simulink model "KinovaBlockdiagram"  (R2022b)
settings: Solver=VariableStepAuto  StartTime=0.0  StopTime=10.0  RelTol=1e-3
undefined symbols (not defined in the file or in its folder): Admittance, forwardKinematics, K, M
settings Model: Creator=KCY  LastModifiedBy=KCY

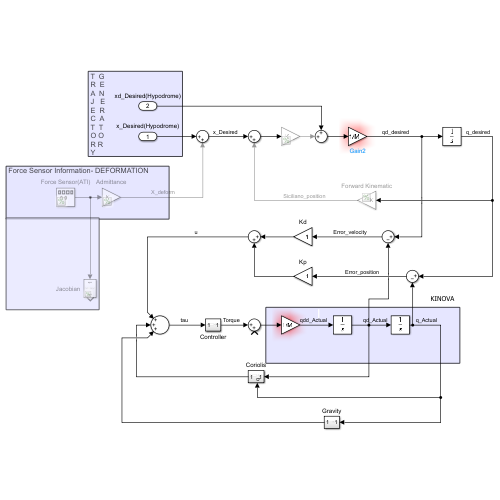
[thumbnail: Simulink's stored preview of the top-level diagram]
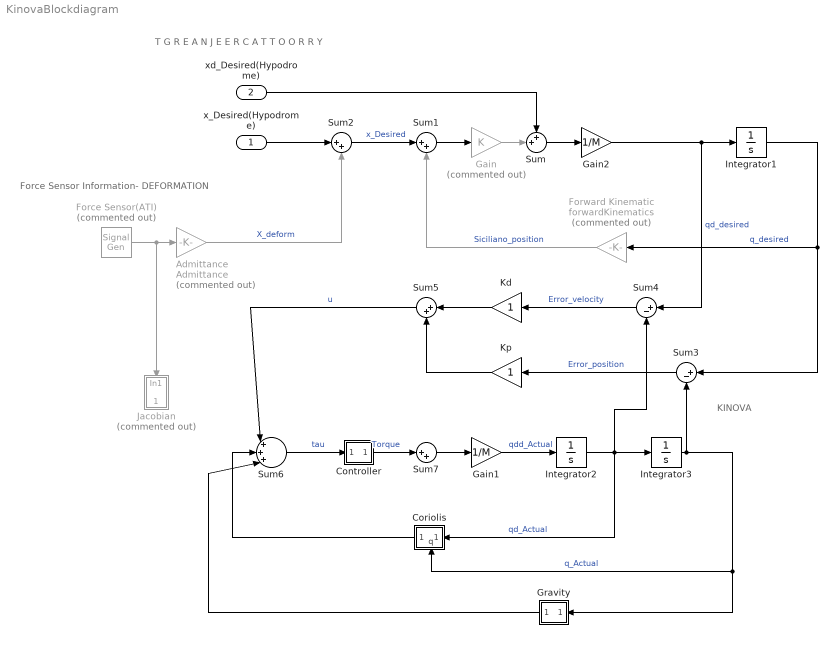
== system KinovaBlockdiagram ==
  note: KINOVA
  note: T  G
      | R  E
      | A  N
      | J   E
      | E  R
      | C  A
      | T  T
      | O O
      | R R
      | Y
  note: Force Sensor Information- DEFORMATION
  x_Desired(Hypodrome) : Inport
  xd_Desired(Hypodrome) : Inport  Port=2
  Admittance : Gain  Commented=on  Gain=Admittance
  Controller : Subsystem
  Coriolis : Subsystem
      settings: PortSchema="{\"entries\":[{\"content\":{\"sides\":[{\"content\":{\"connectorIds\":[\"In1\"]},\"type\":\"ConnectorPlacement.EquallySpacedRectSide\",\"uuid\":\"c197da61-234a-4eb3-9235-43b863a6ed16\"},{\"content\":{\"connectorIds\":[\"Out1\"],\"side\":\"RIGHT\"},\"type\":\"ConnectorPlacement.EquallySpacedRectSide\",\"uuid\":\"0fea028c-9e06-4adc-92e4-6f1c9f077e30\"},{\"content\":{\"connectorIds\":[],\"side\":\"TOP\"},\"type\":\"ConnectorPlacement.EquallySpacedRectSide\",\"uuid\":\"95090893-3b48-409b-94f5-10df5b393291\"},{\"content\":{\"connectorIds\":[\"In2\"],\"side\":\"BOTTOM\"},\"type\":\"ConnectorPlacement.EquallySpacedRectSide\",\"uuid\":\"bf4882cf-b050-4c85-943a-211f52503d2d\"}]},\"type\":\"ConnectorPlacement.EquallySpacedConnector\",\"uuid\":\"e18e85b5-629d-4441-ae51-d53f1b2ec95d\"}],\"packageUris\":[\"http://schema.mathworks.com/mf0/Connector/R2020b\"],\"version\":\"1.0\"}"
  Force Sensor(ATI) : SignalGenerator  Commented=on  Units=rad/sec
  Forward Kinematic : Gain  Commented=on  Gain=forwardKinematics
  Gain : Gain  Commented=on  Gain=K
  Gain1 : Gain  Gain=1/M
  Gain2 : Gain  Gain=1/M
  Gravity : Subsystem
  Integrator1 : Integrator
  Integrator2 : Integrator
  Integrator3 : Integrator
  Jacobian : Subsystem  Commented=on
  Kd : Gain
  Kp : Gain
  Sum : Sum  Inputs=++|
  Sum{1..2,5,7} (4 alike) : Sum  Inputs=|++
  Sum3 : Sum  Inputs=|+-
  Sum4 : Sum  Inputs=|+-
  Sum6 : Sum  Inputs=|+++|
  wires:
  xd_Desired(Hypodrome)/1 -> Sum/1
  Gain/1 -> Sum/2
  x_Desired(Hypodrome)/1 -> Sum2/1
  Sum1/1 -> Gain/1
  Force Sensor(ATI)/1 -> Jacobian/1(In1), Admittance/1
  Admittance/1 -> Sum2/2  "X_deform"
  Sum2/1 -> Sum1/1  "x_Desired"
  Sum/1 -> Gain2/1
  Gain2/1 -> Integrator1/1, Sum4/1  "qd_desired"
  Integrator1/1 -> Sum3/1, Forward Kinematic/1  "q_desired"
  Forward Kinematic/1 -> Sum1/2  "Siciliano_position"
  Sum3/1 -> Kp/1  "Error_position"
  Sum4/1 -> Kd/1  "Error_velocity"
  Kd/1 -> Sum5/1
  Sum5/1 -> Sum6/1  "u"
  Sum6/1 -> Controller/1(In1)  "tau"
  Controller/1(Out1) -> Sum7/1  "Torque"
  Sum7/1 -> Gain1/1
  Gain1/1 -> Integrator2/1  "qdd_Actual"
  Integrator2/1 -> Coriolis/1(In1), Sum4/2, Integrator3/1  "qd_Actual"
  Gravity/1(Out1) -> Sum6/3
  Coriolis/1(Out1) -> Sum6/2
  Integrator3/1 -> Coriolis/2(q), Gravity/1(In1), Sum3/2  "q_Actual"
  Kp/1 -> Sum5/2

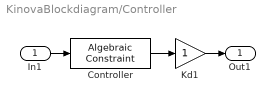
== system KinovaBlockdiagram/Controller ==
  In1 : Inport
  Controller : AlgebraicConstraint  InitialGuess=Controller
  Kd1 : Gain
  Out1 : Outport
  wires:
  Controller/1 -> Kd1/1
  Kd1/1 -> Out1/1
  In1/1 -> Controller/1

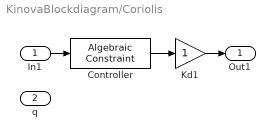
== system KinovaBlockdiagram/Coriolis ==
  In1 : Inport
  q : Inport  Port=2
  Controller : AlgebraicConstraint  InitialGuess=Controller
  Kd1 : Gain
  Out1 : Outport
  wires:
  Controller/1 -> Kd1/1
  Kd1/1 -> Out1/1
  In1/1 -> Controller/1

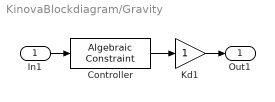
== system KinovaBlockdiagram/Gravity ==
  In1 : Inport
  Controller : AlgebraicConstraint  InitialGuess=Controller
  Kd1 : Gain
  Out1 : Outport
  wires:
  Controller/1 -> Kd1/1
  Kd1/1 -> Out1/1
  In1/1 -> Controller/1

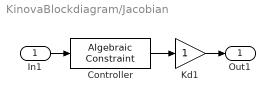
== system KinovaBlockdiagram/Jacobian ==
  In1 : Inport
  Controller : AlgebraicConstraint  InitialGuess=Controller
  Kd1 : Gain
  Out1 : Outport
  wires:
  Controller/1 -> Kd1/1
  Kd1/1 -> Out1/1
  In1/1 -> Controller/1
